simulink subsystem "Day4_5_Scenario_1"  (R2024a)
settings: Solver=VariableStepAuto  StartTime=0.0  StopTime=10.0  RelTol=1e-3
libraries: CarMaker4SL x11
settings Model: Creator=junhyung.cha  LastModifiedBy=pc

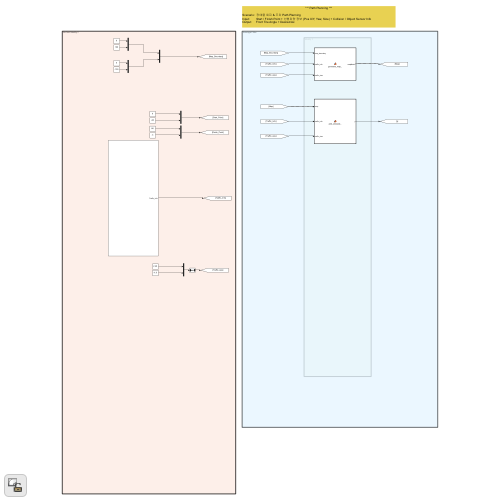
[thumbnail: Simulink's stored preview of the top-level diagram]
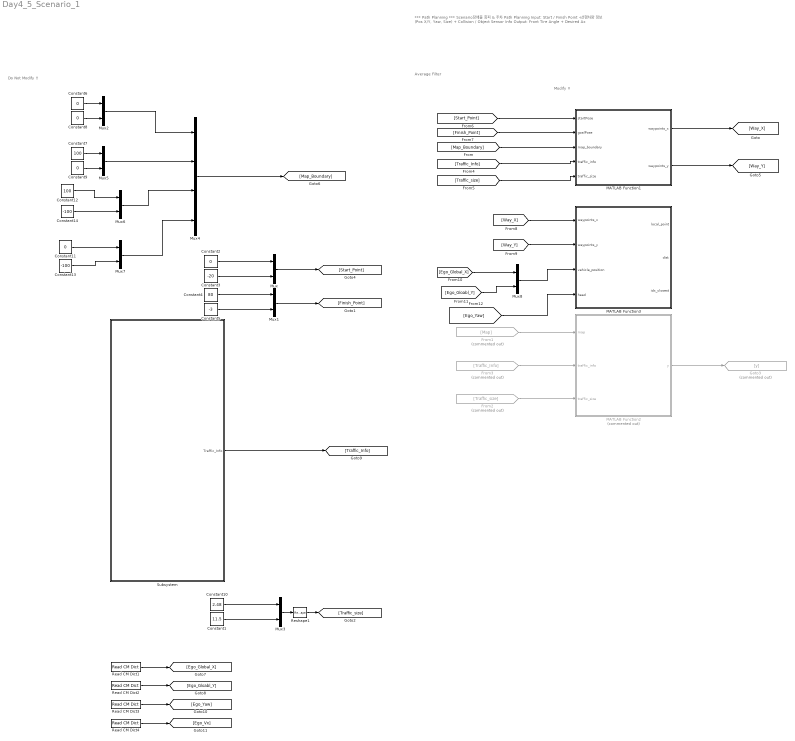
== system Day4_5_Scenario_1 ==
  note: Average Filter
  note: Do Not Modify !!
  note: Modify !!
  note: *** Path Planning ***
      |
      | Scenario: 장애물 회피 & 주차 Path Planning
      | Input: Start / Finish Point + 선행차량 정보 (Pos X/Y, Yaw, Size) + Collision / Object Sensor Info
      | Output: Front Tire Angle + Desired Ax
  Constant1 : Constant  Value=11.5
  Constant10 : Constant  Value=2.48
  Constant{2,6,8..9,11} (5 alike) : Constant  Value=0
  Constant12 : Constant  Value=100
  Constant13 : Constant  Value=-100
  Constant14 : Constant  Value=-100
  Constant3 : Constant  Value=-20
  Constant4 : Constant  Value=80
  Constant5 : Constant  Value=-3
  Constant7 : Constant  Value=100
  From1 : From  Commented=on  GotoTag=Map
  From2 : From  Commented=on  GotoTag=Traffic_size
  From3 : From  Commented=on  GotoTag=Traffic_Info
  Goto3 : Goto  Commented=on  GotoTag=y
  MATLAB Function1 : MATLAB Function  TreatAsAtomicUnit=on
  MATLAB Function2 : MATLAB Function  Commented=on  TreatAsAtomicUnit=on
  MATLAB Function3 : MATLAB Function  TreatAsAtomicUnit=on
  Mux{,1..3,5..8} (8 alike) : Mux  Inputs=2
  Mux4 : Mux
  Read CM Dict1 : CarMaker4SL/Read CM Dict  xname=Car.Fr1.tx  xsync=off  xstime=Inherited
  Read CM Dict2 : CarMaker4SL/Read CM Dict  xname=Car.Fr1.ty  xsync=off  xstime=Inherited
  Read CM Dict3 : CarMaker4SL/Read CM Dict  xname=Car.Fr1.rz  xsync=off  xstime=Inherited
  Read CM Dict4 : CarMaker4SL/Read CM Dict  xname=Car.v  xsync=off  xstime=Inherited
  Reshape1 : Reshape  OutputDimensionality=Row vector (2-D)  OutputDimensions=[2,2]
  Subsystem : Subsystem
  wires:
  From1/1 -> MATLAB Function2/1(map)
  Mux/1 -> [Start_Point]
  Constant2/1 -> Mux/1
  Constant3/1 -> Mux/2
  Constant5/1 -> Mux1/2
  Mux1/1 -> [Finish_Point]
  Constant4/1 -> Mux1/1
  Constant6/1 -> Mux2/1
  Constant8/1 -> Mux2/2
  Constant9/1 -> Mux5/2
  [Map_Boundary] -> MATLAB Function1/3(map_boundary)
  Subsystem/1(Traffic_Info) -> [Traffic_Info]
  From3/1 -> MATLAB Function2/2(traffic_info)
  Mux3/1 -> Reshape1/1
  From2/1 -> MATLAB Function2/3(traffic_size)
  Constant10/1 -> Mux3/1
  Constant1/1 -> Mux3/2
  Mux2/1 -> Mux4/1
  Mux5/1 -> Mux4/2
  Mux4/1 -> [Map_Boundary]
  Constant7/1 -> Mux5/1
  [Traffic_Info] -> MATLAB Function1/4(traffic_info)
  [Traffic_size] -> MATLAB Function1/5(traffic_size)
  Reshape1/1 -> [Traffic_size]
  MATLAB Function1/1(waypoints_x) -> [Way_X]
  MATLAB Function2/1(y) -> Goto3/1
  Constant14/1 -> Mux6/2
  Constant12/1 -> Mux6/1
  Constant11/1 -> Mux7/1
  Constant13/1 -> Mux7/2
  Mux6/1 -> Mux4/3
  Mux7/1 -> Mux4/4
  [Start_Point] -> MATLAB Function1/1(startPose)
  [Finish_Point] -> MATLAB Function1/2(goalPose)
  MATLAB Function1/2(waypoints_y) -> [Way_Y]
  Read CM Dict4/1 -> [Ego_Vx]
  Read CM Dict3/1 -> [Ego_Yaw]
  Read CM Dict1/1 -> [Ego_Global_X]
  Read CM Dict2/1 -> [Ego_Gloabl_Y]
  [Way_Y] -> MATLAB Function3/2(waypoints_y)
  [Way_X] -> MATLAB Function3/1(waypoints_x)
  Mux8/1 -> MATLAB Function3/3(vehicle_position)
  [Ego_Global_X] -> Mux8/1
  [Ego_Gloabl_Y] -> Mux8/2
  [Ego_Yaw] -> MATLAB Function3/4(head)

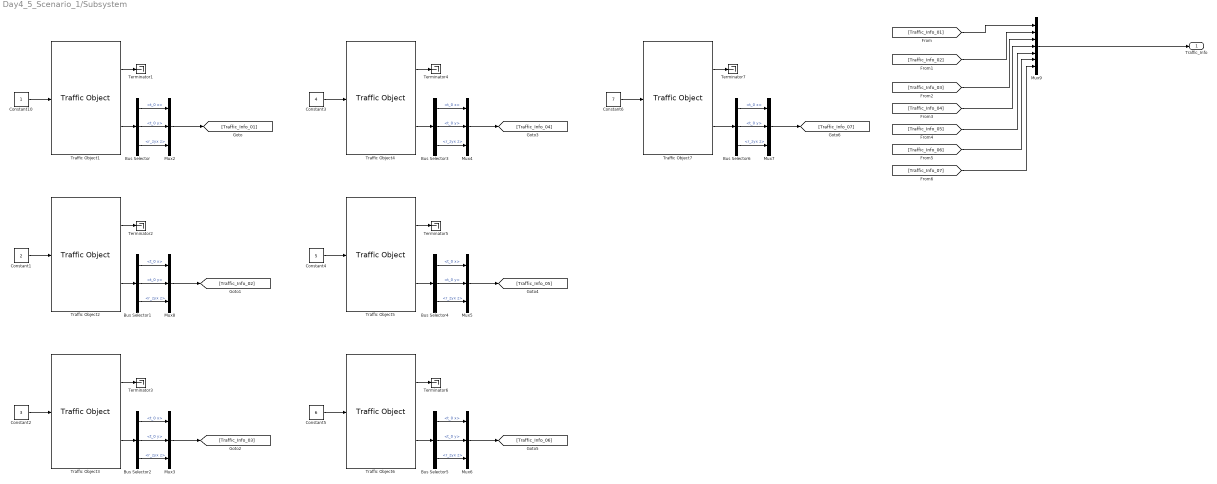
== system Day4_5_Scenario_1/Subsystem ==
  Bus Selector{,1..6} (7 alike) : BusSelector  OutputSignals=t_0 x,t_0 y,r_zyx z
  Constant1 : Constant  Value=2
  Constant10 : Constant
  Constant2 : Constant  Value=3
  Constant3 : Constant  Value=4
  Constant4 : Constant  Value=5
  Constant5 : Constant  Value=6
  Constant6 : Constant  Value=7
  Mux{2..8} (7 alike) : Mux  Inputs=3
  Mux9 : Mux  Inputs=7
  Terminator{1..7} (7 alike) : Terminator
  Traffic Object1 : CarMaker4SL/Traffic Object  xname=T01  ximode=Traffic Id  xstime=Inherited
      settings: SourceProductName=CarMaker4SL
  Traffic Object2 : CarMaker4SL/Traffic Object  xname=T02  ximode=Traffic Id  xstime=Inherited
      settings: SourceProductName=CarMaker4SL
  Traffic Object3 : CarMaker4SL/Traffic Object  xname=T03  ximode=Traffic Id  xstime=Inherited
      settings: SourceProductName=CarMaker4SL
  Traffic Object4 : CarMaker4SL/Traffic Object  xname=T04  ximode=Traffic Id  xstime=Inherited
      settings: SourceProductName=CarMaker4SL
  Traffic Object5 : CarMaker4SL/Traffic Object  xname=T05  ximode=Traffic Id  xstime=Inherited
      settings: SourceProductName=CarMaker4SL
  Traffic Object6 : CarMaker4SL/Traffic Object  xname=T06  ximode=Traffic Id  xstime=Inherited
      settings: SourceProductName=CarMaker4SL
  Traffic Object7 : CarMaker4SL/Traffic Object  xname=T07  ximode=Traffic Id  xstime=Inherited
      settings: SourceProductName=CarMaker4SL
  Traffic_Info : Outport
  wires:
  [Traffic_Info_07] -> Mux9/7
  [Traffic_Info_06] -> Mux9/6
  [Traffic_Info_05] -> Mux9/5
  [Traffic_Info_04] -> Mux9/4
  [Traffic_Info_03] -> Mux9/3
  Mux9/1 -> Traffic_Info/1
  [Traffic_Info_02] -> Mux9/2
  [Traffic_Info_01] -> Mux9/1
  Mux2/1 -> [Traffic_Info_01]
  Traffic Object7/2 -> Bus Selector6/1
  Bus Selector6/3 -> Mux7/3  "<r_zyx z>"
  Bus Selector6/1 -> Mux7/1  "<t_0 x>"
  Mux7/1 -> [Traffic_Info_07]
  Bus Selector6/2 -> Mux7/2  "<t_0 y>"
  Traffic Object6/2 -> Bus Selector5/1
  Bus Selector5/3 -> Mux6/3  "<r_zyx z>"
  Bus Selector5/1 -> Mux6/1  "<t_0 x>"
  Mux6/1 -> [Traffic_Info_06]
  Bus Selector5/2 -> Mux6/2  "<t_0 y>"
  Traffic Object5/2 -> Bus Selector4/1
  Bus Selector4/3 -> Mux5/3  "<r_zyx z>"
  Bus Selector4/1 -> Mux5/1  "<t_0 x>"
  Mux5/1 -> [Traffic_Info_05]
  Bus Selector4/2 -> Mux5/2  "<t_0 y>"
  Traffic Object4/2 -> Bus Selector3/1
  Bus Selector3/3 -> Mux4/3  "<r_zyx z>"
  Bus Selector3/1 -> Mux4/1  "<t_0 x>"
  Mux4/1 -> [Traffic_Info_04]
  Bus Selector3/2 -> Mux4/2  "<t_0 y>"
  Traffic Object3/2 -> Bus Selector2/1
  Bus Selector2/3 -> Mux3/3  "<r_zyx z>"
  Bus Selector2/1 -> Mux3/1  "<t_0 x>"
  Mux3/1 -> [Traffic_Info_03]
  Bus Selector2/2 -> Mux3/2  "<t_0 y>"
  Traffic Object2/2 -> Bus Selector1/1
  Bus Selector1/3 -> Mux8/3  "<r_zyx z>"
  Bus Selector1/1 -> Mux8/1  "<t_0 x>"
  Mux8/1 -> [Traffic_Info_02]
  Bus Selector1/2 -> Mux8/2  "<t_0 y>"
  Bus Selector/3 -> Mux2/3  "<r_zyx z>"
  Bus Selector/2 -> Mux2/2  "<t_0 y>"
  Bus Selector/1 -> Mux2/1  "<t_0 x>"
  Traffic Object1/2 -> Bus Selector/1
  Traffic Object7/1 -> Terminator7/1
  Constant6/1 -> Traffic Object7/1
  Constant5/1 -> Traffic Object6/1
  Traffic Object6/1 -> Terminator6/1
  Traffic Object5/1 -> Terminator5/1
  Constant4/1 -> Traffic Object5/1
  Constant3/1 -> Traffic Object4/1
  Traffic Object4/1 -> Terminator4/1
  Traffic Object3/1 -> Terminator3/1
  Constant2/1 -> Traffic Object3/1
  Constant1/1 -> Traffic Object2/1
  Traffic Object2/1 -> Terminator2/1
  Traffic Object1/1 -> Terminator1/1
  Constant10/1 -> Traffic Object1/1

== matlab function Day4_5_Scenario_1/MATLAB Function3 ==
  settings: sampleTime=0.1
  data: waypoints_x input; local_point output; waypoints_y input; vehicle_position input; head input; dist output; idx_closest output
function [local_point, dist, idx_closest] = global_to_local_waypoints( ...
         waypoints_x, waypoints_y, vehicle_position, head)
%#codegen
% 가장 가까운 글로벌 웨이포인트를 찾아 로컬 좌표 변환
% 추가 출력: idx_closest (현재 선택된 인덱스), N (전체 웨이포인트 수)

    %% 1) 전체 포인트 개수
    N = numel(waypoints_x);

    %% 2) Ego 차량 위치
    X_ego = vehicle_position(1);
    Y_ego = vehicle_position(2);

    %% 3) 모든 웨이포인트와 거리 제곱 계산
    dx_all = waypoints_x - X_ego;     % 1×N
    dy_all = waypoints_y - Y_ego;     % 1×N
    d2_all = dx_all.^2 + dy_all.^2;   % 1×N

    %% 4) 최소 거리인 인덱스 찾기
    [~, idx_closest] = min(d2_all);

    %% 5) 해당 점 로컬 좌표 변환
    gx = waypoints_x(idx_closest);
    gy = waypoints_y(idx_closest);
    c  = cos(-head);
    s  = sin(-head);
    R  = [c, -s; s, c];
    d  = R * ([gx; gy] - [X_ego; Y_ego]);
    local_point = d';                  % 1×2

    %% 6) 실제 거리 계산
    dist = sqrt(d2_all(idx_closest));  % 스칼라
end

== matlab function Day4_5_Scenario_1/MATLAB Function1 ==
  settings: sampleTime=0.05
  data: startPose input; goalPose input; map_boundary input; waypoints_x output size=[1000, 1000]; traffic_info input; traffic_size input; waypoints_y output
function [waypoints_x, waypoints_y] = rrt_star_block(startPose, goalPose, map_boundary, traffic_info, traffic_size)
%#codegen
% RRT* planner for Simulink MATLAB Function block
% Inputs:
%   startPose      : [1x2] [x y]
%   goalPose       : [1x2] [x y]
%   map_boundary   : [1x8] [x1 y1 x2 y2 ...]
%   traffic_info   : [Nx3] [x y yaw]
%   traffic_size   : [Nx2] [width height]
% Outputs:
%   waypoints_x    : Mx1 vector of x-coordinates of final path
%   waypoints_y    : Mx1 vector of y-coordinates of final path

    %% Parameters
    maxIter        = 5000;
    stepSize       = 2;
    goalSampleRate = 0.1;
    successDistTh  = 5;
    collisionRes   = 0.5;
    searchRadius   = 10;
    safetyDist     = 2;
    maxNodes       = maxIter + 1;

    %% Generate occupancy map
    map = generate_map_1(map_boundary, traffic_info, traffic_size);
    [mapH, mapW] = size(map);

    %% Preallocate node arrays
    nodes_x   = zeros(maxNodes,1);
    nodes_y   = zeros(maxNodes,1);
    parent    = zeros(maxNodes,1);
    cost_arr  = inf(maxNodes,1);

    %% Initialize tree
    nodes_x(1)  = startPose(1);
    nodes_y(1)  = startPose(2);
    parent(1)   = 0;
    cost_arr(1) = 0;
    nodeCount   = 1;
    goalReached = false;

    %% Main RRT* loop
    for iter = 1:maxIter
        % Sample random point
        if rand < goalSampleRate
            xr = goalPose;
        else
            xr = [1 + floor(rand*(mapW-1)), 1 + floor(rand*(mapH-1))];
        end

        % Nearest node
        [nearestIdx] = findNearest(nodes_x, nodes_y, nodeCount, xr);
        nearXY = [nodes_x(nearestIdx), nodes_y(nearestIdx)];

        % Steer
        theta = atan2(xr(2)-nearXY(2), xr(1)-nearXY(1));
        newXY = nearXY + stepSize * [cos(theta), sin(theta)];

        % Collision & safety check
        if isCollision(newXY, map) || isPathCollision(nearXY, newXY, map, collisionRes) || isNearObstacle(newXY, map, safetyDist)
            continue;
        end

        % Find neighbors
        nearIdxs = findNearNodes(nodes_x, nodes_y, nodeCount, newXY, searchRadius);

        % Choose best parent
        minCost   = cost_arr(nearestIdx) + norm(newXY - nearXY);
        minParent = nearestIdx;
        for j = 1:numel(nearIdxs)
            i = nearIdxs(j);
            pxy = [nodes_x(i), nodes_y(i)];
            if ~isPathCollision(pxy, newXY, map, collisionRes)
                c = cost_arr(i) + norm(newXY - pxy);
                if c < minCost
                    minCost   = c;
                    minParent = i;
                end
            end
        end

        % Add new node
        nodeCount = nodeCount + 1;
        nodes_x(nodeCount)  = newXY(1);
        nodes_y(nodeCount)  = newXY(2);
        parent(nodeCount)   = minParent;
        cost_arr(nodeCount)= minCost;

        % Rewire
        for j = 1:numel(nearIdxs)
            i = nearIdxs(j);
            pxy = [nodes_x(i), nodes_y(i)];
            c = minCost + norm([newXY(1), newXY(2)] - pxy);
            if c < cost_arr(i) && ~isPathCollision(newXY, pxy, map, collisionRes)
                parent(i)    = nodeCount;
                cost_arr(i)  = c;
            end
        end

        % Check goal reach
        if norm(newXY - goalPose) < successDistTh
            goalReached = true;
            lastIdx = nodeCount;
            break;
        end
    end

    %% Backtrace path
    if goalReached
        % Count backward
        tmpIdx = lastIdx;
        M = 0;
        while tmpIdx ~= 0 && M < maxNodes
            M = M + 1;
            way_x(M) = nodes_x(tmpIdx); %#ok<AGROW>
            way_y(M) = nodes_y(tmpIdx); %#ok<AGROW>
            tmpIdx = parent(tmpIdx);
        end
        % Reverse order
        waypoints_x = way_x(M:-1:1)';
        waypoints_y = way_y(M:-1:1)';
    else
        waypoints_x = zeros(0,1);
        waypoints_y = zeros(0,1);
    end
end

%%% Helper functions %%%
function mapMatrix = generate_map_1(map_boundary, traffic_info, traffic_size)
    resolution = 1;
    xs = map_boundary(1:2:end);
    ys = map_boundary(2:2:end);
    x_min = min(xs); x_max = max(xs);
    y_min = min(ys); y_max = max(ys);
    W = ceil((x_max-x_min)/resolution);
    H = ceil((y_max-y_min)/resolution);
    mapMatrix = zeros(H, W);
    N = min(size(traffic_info,1), size(traffic_size,1));
    for i=1:N
        x_c = traffic_info(i,1);
        y_c = traffic_info(i,2);
        yaw = traffic_info(i,3);
        w = traffic_size(i,1);
        h = traffic_size(i,2);
        % Define corners
        dx = w/2; dy = h/2;
        local = [-dx,-dy; dx,-dy; dx,dy; -dx,dy];
        R = [cos(yaw), -sin(yaw); sin(yaw), cos(yaw)];
        corners = (R*local')';
        center = [x_c, y_c] + (w/2)*[cos(yaw), sin(yaw)] - (h/2)*[-sin(yaw), cos(yaw)];
        corners = corners + center;
        xi = (corners(:,1)-x_min)/resolution + 1;
        yi = (y_max-corners(:,2))/resolution + 1;
        mask = poly2mask(xi, yi, H, W);
        mapMatrix(mask) = 1;
    end
end

function idx = findNearest(nx, ny, N, sample)
    dmin = inf;
    idx  = 1;
    for k=1:N
        d = hypot(nx(k)-sample(1), ny(k)-sample(2));
        if d < dmin
            dmin = d;
            idx  = k;
        end
    end
end

function nearIdxs = findNearNodes(nx, ny, N, pos, R)
    count = 0;
    nearIdxs = zeros(N,1);
    for k=1:N
        if hypot(nx(k)-pos(1), ny(k)-pos(2)) <= R
            count = count + 1;
            nearIdxs(count) = k;
        end
    end
    nearIdxs = nearIdxs(1:count);
end

function flag = isCollision(pt, map)
    x = round(pt(1)); y = round(pt(2));
    if x<1||x>size(map,2)||y<1||y>size(map,1)
        flag = true;
    else
        flag = (map(y,x)==1);
    end
end

function flag = isPathCollision(p1, p2, map, step)
    d = hypot(p2(1)-p1(1), p2(2)-p1(2));
    N = max(1, ceil(d/step));
    flag = false;
    for i=0:N
        pt = p1 + (p2-p1)*(i/N);
        if isCollision(pt, map)
            flag = true; return;
        end
    end
end

function flag = isNearObstacle(pt, map, sd)
    x0 = round(pt(1)); y0 = round(pt(2));
    r  = ceil(sd);
    [X,Y] = meshgrid(x0-r:x0+r, y0-r:y0+r);
    D2 = (X-pt(1)).^2 + (Y-pt(2)).^2;
    mask = (D2 <= sd^2);
    X = X(mask); Y = Y(mask);
    valid = X>=1 & X<=size(map,2) & Y>=1 & Y<=size(map,1);
    X = X(valid); Y = Y(valid);
    flag = any(map(sub2ind(size(map), Y, X))==1);
end

== matlab function Day4_5_Scenario_1/MATLAB Function2 ==
  settings: sampleTime=0.1
  data: map input; y output; traffic_info input; traffic_size input
function y = add_obstacle_(map, traffic_info, traffic_size)
    y = 0;
end
